simulink model "REAL_TIME_TRACKING"  (R2024b)
settings: Solver=ode4  StartTime=0.0  StopTime=T_SIM  FixedStep=T_s  RelTol=1e-3
undefined symbols (not defined in the file): control_par, controller_index, d, D, d_actual, H_enc, H_gyro, H_motion_cap, omega_M, omega_max, P_INIT_EKF, p_loss, PHI_INIT, Q_INIT, Q_INIT_LOC, r, R_3, r_actual, state_type, T_s, T_trj, trj_index, X, Y, Z_INIT_EKF
libraries: robotlib x6, sharedtransform x1
settings Model: Creator=llp  LastModifiedBy=tomailoren
settings OptimizationCC: DefaultParameterBehavior=Inlined  EnhancedBackFolding=on  PassReuseOutputArgsAs=Individual arguments  ZeroExternalMemoryAtStartup=off  ZeroInternalMemoryAtStartup=off  MaxStackSize=64  OptimizeBlockOrder=speed  DifferentSizesBufferReuse=on  OptimizationCustomize=off  EfficientTunableParamExpr=on
settings DebuggingCC: ParameterTunabilityLossMsg=error
settings SFSimCC: MATLABDynamicMemAlloc=off
settings RTWCC: Description=Embedded Coder  SystemTargetFile=ert.tlc  HardwareBoard=Robot Operating System 2 (ROS 2)  TLCOptions="-aInlineSetEventsForThisBaseRateFcn=TLC_FALSE -aSuppressMultiTaskScheduler=TLC_FALSE  -aRateBasedStepFcn=0"  TemplateMakefile=ert_default_tmf  Toolchain=Colcon Tools  TargetLang=C++
settings CodeAppCC: ForceParamTrailComments=on  IgnoreCustomStorageClasses=off  OperatorAnnotations=on  SimulinkDataObjDesc=on  SFDataObjDesc=on  InsertBlockDesc=on
settings ERTTargetCC: CodeInterfacePackaging=C++ class  RootIOFormat=Structure reference

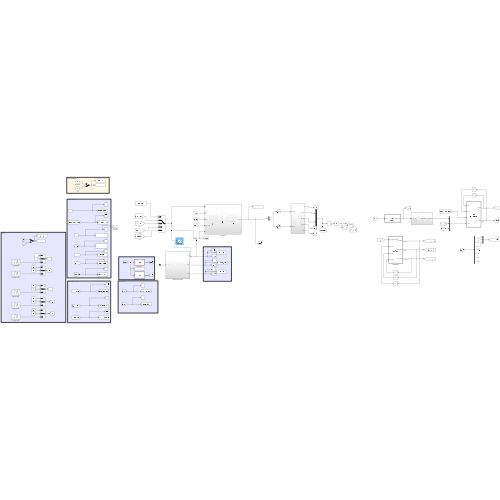
[thumbnail: Simulink's stored preview of the top-level diagram]
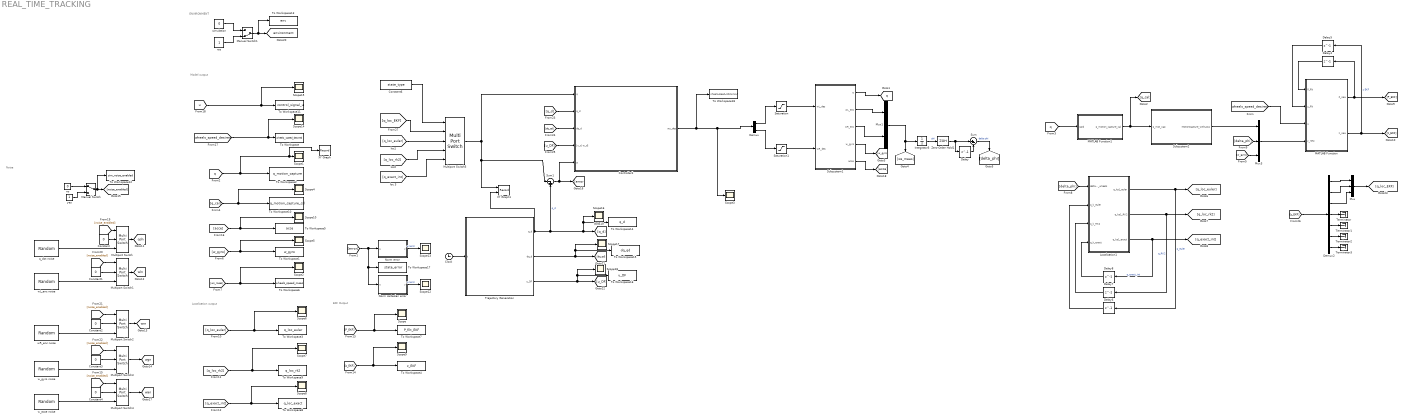
== system REAL_TIME_TRACKING ==
  note: Noise
  note: Localization output
  note: EKF Output
  note: Model output
  note: ENVIRONMENT
  Clock : Clock
  Constant{,1..4} (5 alike) : Constant  Value=0
  Constant6 : Constant  Value=state_type
  Controller1 : Subsystem
  Delay : Delay  DelayLength=1  InitialCondition=[0;0]  SampleTime=T_s
  Delay4 : Delay  DelayLength=1  InitialCondition=P_INIT_EKF  SampleTime=T_s
  Delay5 : Delay  DelayLength=1  InitialCondition=Z_INIT_EKF  SampleTime=T_s
  Delay6 : Delay  DelayLength=1  InitialCondition=Q_INIT_LOC
  Delay7 : Delay  DelayLength=1  InitialCondition=Q_INIT_LOC
  Delay8 : Delay  DelayLength=1  InitialCondition=Q_INIT_LOC
  Demux : Demux  Outputs=2
  Demux2 : Demux  Outputs=7
  Integrator5 : Integrator  InitialCondition=PHI_INIT
  Localization1 : MATLAB Function  TreatAsAtomicUnit=on
  MATLAB Function : MATLAB Function  TreatAsAtomicUnit=on
  MATLAB Function1 : MATLAB Function  TreatAsAtomicUnit=on
  Manual Switch : ManualSwitch
  Manual Switch1 : ManualSwitch  CurrentSetting=0
  Multiport Switch{,1..4} (5 alike) : MultiPortSwitch  DataPortOrder=Zero-based contiguous  Inputs=2  zeroidx=on  SaturateOnIntegerOverflow=off  InputSameDT=off
  Multiport Switch5 : MultiPortSwitch  Inputs=4  SaturateOnIntegerOverflow=off  InputSameDT=off
  Mux : Mux  Inputs=3
  Mux1 : Mux  Inputs=2
  Mux3 : Mux  Inputs=3
  Norm cartesian error : MATLAB Function  TreatAsAtomicUnit=on
  Norm error : MATLAB Function  TreatAsAtomicUnit=on
  Saturation : Saturate  UpperLimit=omega_max  LowerLimit=-omega_max
  Saturation1 : Saturate  UpperLimit=omega_max  LowerLimit=-omega_max
  Scope{,1..10,12..18} (18 alike) : Scope
  Subsystem1 : Subsystem
  Subsystem2 : Subsystem
  Sum : Sum  Inputs=|+-
  Sum1 : Sum  Inputs=|-+
  Terminator{,1..3} (4 alike) : Terminator
  To Workspace : ToWorkspace  VariableName=wheels_speed_desired  SaveFormat=Structure With Time  SampleTime=-1
  To Workspace1 : ToWorkspace  VariableName=w_gyro  SaveFormat=Structure With Time  SampleTime=-1
  To Workspace10 : ToWorkspace  VariableName=q_motion_capture_cal  SaveFormat=Structure With Time  SampleTime=-1
  To Workspace11 : ToWorkspace  VariableName=control_signal_u  SaveFormat=Timeseries  SampleTime=-1
  To Workspace12 : ToWorkspace  VariableName=sim_noise_enabled  SaveFormat=Structure  SampleTime=-1
      settings: Save2DSignal=2-D array (concatenate along first dimension)
  To Workspace13 : ToWorkspace  VariableName=env  SaveFormat=Structure  SampleTime=-1
      settings: Save2DSignal=2-D array (concatenate along first dimension)
  To Workspace14 : ToWorkspace  VariableName=q_d  SaveFormat=Structure With Time  SampleTime=-1
  To Workspace15 : ToWorkspace  VariableName=dq_qd  SaveFormat=Structure With Time  SampleTime=-1
  To Workspace16 : ToWorkspace  VariableName=u_DF  SaveFormat=Structure With Time  SampleTime=-1
  To Workspace17 : ToWorkspace  VariableName=state_error  SaveFormat=Structure With Time  SampleTime=-1
  To Workspace18 : ToWorkspace  VariableName=wheels_speed_robot_input  SaveFormat=Structure With Time  SampleTime=-1
  To Workspace2 : ToWorkspace  VariableName=q_motion_capture  SaveFormat=Structure With Time  SampleTime=-1
  To Workspace3 : ToWorkspace  VariableName=q_loc_euler  SaveFormat=Structure With Time  SampleTime=-1
  To Workspace4 : ToWorkspace  VariableName=z_EKF  SaveFormat=Structure With Time  SampleTime=-1
  To Workspace5 : ToWorkspace  VariableName=acce  SaveFormat=Structure With Time  SampleTime=-1
  To Workspace6 : ToWorkspace  VariableName=wheels_speed_meas  SaveFormat=Structure With Time  SampleTime=-1
  To Workspace7 : ToWorkspace  VariableName=P_filt_EKF  SaveFormat=Structure With Time  SampleTime=-1
  To Workspace8 : ToWorkspace  VariableName=q_loc_exact  SaveFormat=Structure With Time  SampleTime=-1
  To Workspace9 : ToWorkspace  VariableName=q_loc_rk2  SaveFormat=Structure With Time  SampleTime=-1
  Trajectory Generation : Subsystem
  XY Graph : Record  FileSettingsInternal="{\"entries\":[{\"content\":{\"excelSettings\":{\"content\":{},\"type\":\"Streamout.ExcelSettings\"}},\"type\":\"Streamout.FileSettingStorage\",\"uuid\":\"\"}],\"packageUris\":[\"http:\\/\\/schema.mathworks.com\\/mf0\\/streamout_blocks\\/R2020a\"],\"version\":\"1.0\"}"  Layout=[1 1]  SignalsInternal="{\"entries\":[{\"content\":{\"signals\":[{\"content\":{\"blockPath\":[],\"dimensions\":[3,1],\"domain\":\"\",\"hasChildren\":true,\"lineColor\":\"#4dbeee\",\"lineWidth\":2,\"port\":1,\"sid\":[\"\"],\"signalID\":1,\"signalName\":\"From2\"},\"type\":\"RecordBlkView.Signal\",\"uuid\":\"\"},{\"content\":{\"blockPath\":[],\"channel\":[1,1],\"dimensions\":[3,1],\"domain\":\"\",\"lineColor\":\"#77ac30\",\"lineWidth\":2,\"parentID\":1,\"port\":1,\"sid\":[\"\"],\"signalID\":2,\"signalName\":\"From2\"},\"type\":\"RecordBlkView.Signal\",\"uuid\":\"\"},{\"content\":{\"blockPath\":[],\"channel\":[2,1],\"dimensions\":[3,1],\"domain\":\"\",\"lineColor\":\"#fe330a\",\"lineWidth\":2,\"parentID\":1,\"port\":1,\"sid\":[\"\"],\"signalID\":3,\"signalName\":\"From2\"},\"type\":\"RecordBlkView.Signal\",\"uuid\":\"\"},{\"content\":{\"blockPath\":[],\"channel\":[3,1],\"dimensions\":[3,1],\"domain\":\"\",\"lineColor\":\"#22b573\",\"lineWidth\":2,\"parentID\":1,\"port\":1,\"sid\":[\"\"],\"signalID\":4,\"signalName\":\"From2\"},\"type\":\"RecordBlkView.Signal\",\"uuid\":\"\"}]},\"type\":\"RecordBlkView.InputSignals\",\"uuid\":\"\"}],\"packageUris\":[\"http:\\/\\/schema.mathworks.com\\/mf0\\/streamout_blocks\\/R2020a\"],\"version\":\"1.0\"}"  VisualizationBindings="{\"xyplotplugin\":{\"info\":[{\"series\":[],\"subplotID\":1}]}}"  CompatibilityTag=XY
  XY Graph1 : Record  FileSettingsInternal="{\"entries\":[{\"content\":{\"excelSettings\":{\"content\":{},\"type\":\"Streamout.ExcelSettings\"}},\"type\":\"Streamout.FileSettingStorage\",\"uuid\":\"\"}],\"packageUris\":[\"http:\\/\\/schema.mathworks.com\\/mf0\\/streamout_blocks\\/R2020a\"],\"version\":\"1.0\"}"  Layout=[1 1]  SignalsInternal="{\"entries\":[{\"content\":{\"signals\":[{\"content\":{\"blockPath\":[],\"dimensions\":[3,1],\"domain\":\"\",\"hasChildren\":true,\"lineColor\":\"#0072bd\",\"lineWidth\":2,\"port\":1,\"sid\":[\"\"],\"signalID\":1,\"signalName\":\"Multiport\\nSwitch5\"},\"type\":\"RecordBlkView.Signal\",\"uuid\":\"\"},{\"content\":{\"blockPath\":[],\"channel\":[1,1],\"dimensions\":[3,1],\"domain\":\"\",\"lineColor\":\"#0072bd\",\"lineWidth\":2,\"parentID\":1,\"plots\":[ 1 ],\"port\":1,\"sid\":[\"\"],\"signalID\":2,\"signalName\":\"Multiport\\nSwitch5\"},\"type\":\"RecordBlkView.Signal\",\"uuid\":\"\"},{\"content\":{\"blockPath\":[],\"dimensions\":[3,1],\"domain\":\"\",\"hasChildren\":true,\"lineColor\":\"#edb120\",\"lineWidth\":2,\"port\":2,\"sid\":[\"\"],\"signalID\":3,\"signalName\":\"q_d\"},\"type\":\"RecordBlkView.Signal\",\"uuid\":\"\"},{\"content\":{\"blockPath\":[],\"channel\":[1,1],\"dimensions\":[3,1],\"domain\":\"\",\"lineColor\":\"#d95319\",\"lineWidth\":2,\"parentID\":3,\"plots\":[ 1 ],\"port\":2,\"sid\":[\"\"],\"signalID\":4,\"signalName\":\"q_d\"},\"type\":\"RecordBlkView.Signal\",\"uuid\":\"\"},{\"content\":{\"blockPath\":[],\"channel\":[2,1],\"dimensions\":[3,1],\"domain\":\"\",\"lineColor\":\"#0072bd\",\"lineWidth\":2,\"parentID\":1,\"plots\":[ 1 ],\"port\":1,\"sid\":[\"\"],\"signalID\":5,\"signalName\":\"Multiport\\nSwitch5\"},\"type\":\"RecordBlkView.Signal\",\"uuid\":\"\"},{\"content\":{\"blockPath\":[],\"channel\":[3,1],\"dimensions\":[3,1],\"domain\":\"\",\"lineColor\":\"#ff13a6\",\"lineWidth\":2,\"parentID\":1,\"port\":1,\"sid\":[\"\"],\"signalID\":6,\"signalName\":\"Multiport\\nSwitch5\"},\"type\":\"RecordBlkView.Signal\",\"uuid\":\"\"},{\"content\":{\"blockPath\":[],\"channel\":[2,1],\"dimensions\":[3,1],\"domain\":\"\",\"lineColor\":\"#fe330a\",\"lineWidth\":2,\"parentID\":3,\"plots\":[ 1 ],\"port\":2,\"sid\":[\"\"],\"signalID\":7,\"signalName\":\"q_d\"},\"type\":\"RecordBlkView.Signal\",\"uuid\":\"\"},{\"content\":{\"blockPath\":[],\"channel\":[3,1],\"dimensions\":[3,1],\"domain\":\"\",\"lineColor\":\"#22b573\",\"lineWidth\":2,\"parentID\":3,\"port\":2,\"sid\":[\"\"],\"signalID\":8,\"signalName\":\"q_d\"},\"type\":\"RecordBlkView.Signal\",\"uuid\":\"\"}]},\"type\":\"RecordBlkView.InputSignals\",\"uuid\":\"\"}],\"packageUris\":[\"http:\\/\\/schema.mathworks.com\\/mf0\\/streamout_blocks\\/R2020a\"],\"version\":\"1.0\"}"  VisualizationBindings="{\"xyplotplugin\":{\"info\":[{\"series\":[{\"bindingParametersList\":[{\"parameter\":\"X-Axis\",\"signalID\":4,\"signalName\":\"q_d(1,1)\"},{\"parameter\":\"Y-Axis\",\"signalID\":7,\"signalName\":\"q_d(2,1)\"}],\"seriesID\":0},{\"bindingParametersList\":[{\"parameter\":\"X-Axis\",\"signalID\":2,\"signalName\":\"Multiport\\nSwitch5(1,1)\"},{\"parameter\":\"Y-Axis\",\"signalID\":5,\"signalName\":\"Multiport\\nSwitch5(2,1)\"}],\"seriesID\":1}],\"subplotID\":1}]}}"  CompatibilityTag=XY
  Zero-Order Hold1 : ZeroOrderHold  SampleTime=T_s
  no : Constant  Value=0
  q_dot noise : RandomNumber  Variance=0.01  SampleTime=T_s
  ros : Constant
  simulation : Constant  Value=0
  wL_enc noise : RandomNumber  Variance=0.01  Seed=1  SampleTime=T_s
  wR_enc noise : RandomNumber  Variance=0.01  Seed=2  SampleTime=T_s
  w_acce noise : RandomNumber  Variance=0.01  Seed=3  SampleTime=T_s
  w_gyro noise : RandomNumber  Variance=0.01  Seed=3  SampleTime=T_s
  yes : Constant
  tag scope: environment=global, q=global, qdn=global, wan=global, wgn=global, wln=global, wrn=global
  wires:
  [z_EKF] -> Scope9/1, To Workspace4/1
  [error] -> To Workspace17/1, Norm cartesian error/1(u), Norm error/1(u)
  simulation/1 -> Manual Switch1/1
  q_dot noise/1 -> Multiport Switch/3
  Integrator5/1 -> Zero-Order Hold1/1  "phi"
  [u] -> Scope15/1, To Workspace11/1
  [noise_enabled] -> Multiport Switch2/1
  Zero-Order Hold1/1 -> Delay/1, Sum/1
  [q_loc_rk2] -> Scope7/1, To Workspace9/1
  [wheels_speed_desired] -> Scope14/1, To Workspace/1
  Subsystem1/3(wR_enc) -> Mux1/2
  Norm cartesian error/1(y) -> Scope12/1  "p norm"
  [q] -> MATLAB Function1/1(q4id)
  Sum1/1 -> Controller1/5(e), [error]
  Norm error/1(y) -> Scope13/1  "e norm"
  Manual Switch/1 -> To Workspace12/1, [noise_enabled]
  Constant3/1 -> Multiport Switch3/2
  Saturation1/1 -> Subsystem1/2(wR_des)
  Delay/1 -> Sum/2
  [noise_enabled] -> Multiport Switch3/1
  wR_enc noise/1 -> Multiport Switch2/3
  ros/1 -> Manual Switch1/2
  Sum/1 -> [delta_phi]  "delta phi"
  Multiport Switch2/1 -> [wrn]
  Multiport Switch/1 -> [qdn]
  Demux/2 -> Saturation1/1
  Subsystem1/2(wL_enc) -> Mux1/1
  Mux1/1 -> Integrator5/1, [ws_meas]
  no/1 -> Manual Switch/1
  Subsystem1/5(acce) -> [acce]
  Subsystem1/4(w_gyro) -> [w_gyro]
  [P_EKF] -> Scope/1, To Workspace7/1
  [delta_phi] -> Localization1/1(delta_angles_wheels)
  Subsystem1/1(q) -> [q]
  w_gyro noise/1 -> Multiport Switch3/3
  Constant4/1 -> Multiport Switch4/2
  [q_exact_int] -> Scope8/1, To Workspace8/1
  [q_loc_euler] -> Scope6/1, To Workspace3/1
  [acce] -> Scope10/1, To Workspace5/1
  Multiport Switch1/1 -> [wln]
  w_acce noise/1 -> Multiport Switch4/3
  [noise_enabled] -> Multiport Switch4/1
  [noise_enabled] -> Multiport Switch/1
  [q_cal] -> To Workspace10/1, Scope4/1
  Constant/1 -> Multiport Switch/2
  yes/1 -> Manual Switch/2
  [q] -> XY Graph/1, Scope1/1, To Workspace2/1
  Constant2/1 -> Multiport Switch2/2
  wL_enc noise/1 -> Multiport Switch1/3
  Demux/1 -> Saturation/1
  Multiport Switch3/1 -> [wgn]
  [ws_meas] -> Scope2/1, To Workspace6/1
  [noise_enabled] -> Multiport Switch1/1
  Constant1/1 -> Multiport Switch1/2
  Multiport Switch4/1 -> [wan]
  MATLAB Function1/1(q_motion_capture_cal) -> [q_cal], Subsystem2/1(q_mot_cap)
  [w_gyro] -> Scope5/1, To Workspace1/1
  Saturation/1 -> Subsystem1/1(wL_des)
  Localization1/3(q_kp1_exact) -> [q_exact_int], Delay8/1  "q_exact_int"
  [w_gyro] -> Mux3/3
  [delta_phi] -> Mux3/2
  MATLAB Function/1(P_new) -> [P_EKF], Delay4/1
  Delay5/1 -> MATLAB Function/2(z_filt)
  Delay4/1 -> MATLAB Function/1(P_filt)
  Manual Switch1/1 -> [environment], To Workspace13/1
  MATLAB Function/2(z_new) -> [z_EKF], Delay5/1  "z EKF"
  Mux3/1 -> MATLAB Function/4(y_new)
  [wheels_speed_desired] -> MATLAB Function/3(u)
  Delay6/1 -> Localization1/2(q_k_euler)
  Delay8/1 -> Localization1/4(q_k_exact)
  Localization1/1(q_kp1_euler) -> [q_loc_euler], Delay6/1  "q_euler"
  Localization1/2(q_kp1_RK2) -> [q_loc_rk2], Delay7/1  "q_RK2"
  Constant6/1 -> Multiport Switch5/1
  Delay7/1 -> Localization1/3(q_k_RK2)
  Subsystem2/1(MotionCapture_withLoss) -> Mux3/1
  [q_loc_EKF] -> Multiport Switch5/2
  [q_loc_euler] -> Multiport Switch5/3
  Trajectory Generation/1(q_d) -> XY Graph1/2, Sum1/2, Scope16/1, To Workspace14/1, [q_d]  "q_d"
  [q_d] -> Controller1/2(q_d)
  [dq_qd] -> Controller1/3(dq_d)
  [u_DF] -> Controller1/4("[v_d, w_d]")
  Trajectory Generation/2(dq_d) -> To Workspace15/1, Scope17/1, [dq_qd]
  Trajectory Generation/3(u_DF) -> To Workspace16/1, Scope18/1, [u_DF]
  Clock/1 -> Trajectory Generation/1(t)
  Controller1/1(ws_des) -> To Workspace18/1, Demux/1, Scope3/1
  [z_EKF] -> Demux2/1
  Demux2/1 -> Mux/1
  Demux2/2 -> Mux/2
  Demux2/3 -> Mux/3
  Mux/1 -> [q_loc_EKF]
  Demux2/4 -> Terminator/1
  Demux2/5 -> Terminator1/1
  Demux2/6 -> Terminator2/1
  Demux2/7 -> Terminator3/1
  [q_loc_rk2] -> Multiport Switch5/4
  [q_exact_int] -> Multiport Switch5/5
  Multiport Switch5/1 -> Controller1/1(q), XY Graph1/1, Sum1/1

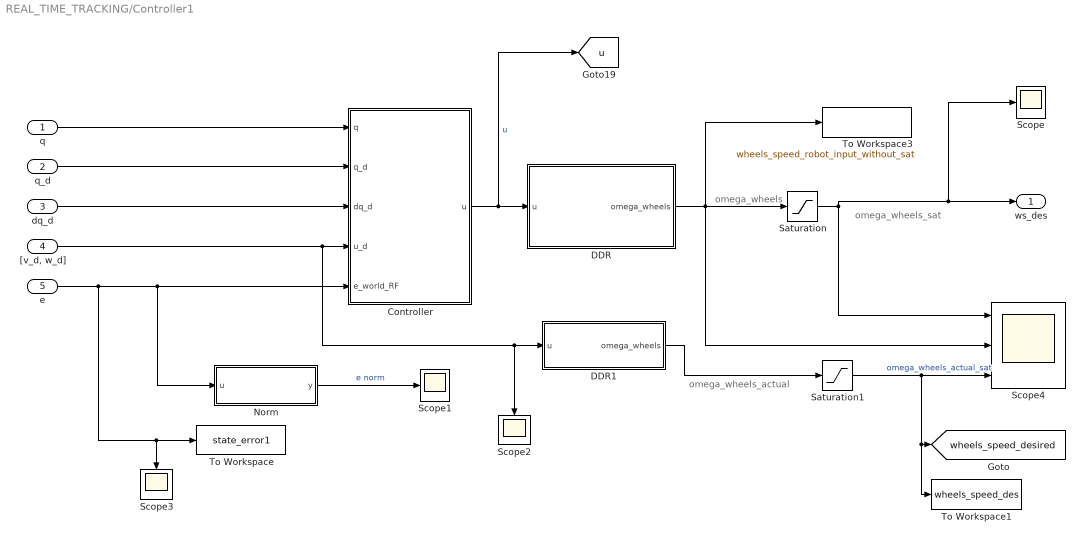
== system REAL_TIME_TRACKING/Controller1 ==
  note: omega_wheels_actual
  note: omega_wheels_sat
  note: omega_wheels
  q : Inport
  q_d : Inport  Port=2
  dq_d : Inport  Port=3
  "[v_d, w_d]" : Inport  Port=4
  e : Inport  Port=5
  Controller : MATLAB Function  TreatAsAtomicUnit=on
  DDR : MATLAB Function  TreatAsAtomicUnit=on
  DDR1 : MATLAB Function  TreatAsAtomicUnit=on
  Norm : MATLAB Function  TreatAsAtomicUnit=on
  Saturation : Saturate  UpperLimit=omega_M  LowerLimit=-omega_M
  Saturation1 : Saturate  UpperLimit=omega_M  LowerLimit=-omega_M
  Scope{,1..3} (4 alike) : Scope
  Scope4 : Scope  NumInputPorts=3
  To Workspace : ToWorkspace  VariableName=state_error1  SaveFormat=Structure With Time  SampleTime=-1
  To Workspace1 : ToWorkspace  VariableName=wheels_speed_des  SaveFormat=Structure With Time  SampleTime=-1
  To Workspace3 : ToWorkspace  VariableName=wheels_speed_robot_input_without_sat  SaveFormat=Structure With Time  SampleTime=-1
  ws_des : Outport
  tag scope: u=global, wheels_speed_desired=global
  wires:
  Saturation/1 -> Scope4/1, Scope/1, ws_des/1
  Saturation1/1 -> To Workspace1/1, [wheels_speed_desired], Scope4/3  "omega_wheels_actual_sat"
  DDR1/1(omega_wheels) -> Saturation1/1
  DDR/1(omega_wheels) -> To Workspace3/1, Scope4/2, Saturation/1
  q/1 -> Controller/1(q)
  dq_d/1 -> Controller/3(dq_d)
  Norm/1(y) -> Scope1/1  "e norm"
  q_d/1 -> Controller/2(q_d)
  e/1 -> Controller/5(e_world_RF), Norm/1(u), Scope3/1, To Workspace/1
  "[v_d, w_d]"/1 -> DDR1/1(u), Scope2/1, Controller/4(u_d)
  Controller/1(u) -> [u], DDR/1(u)  "u"

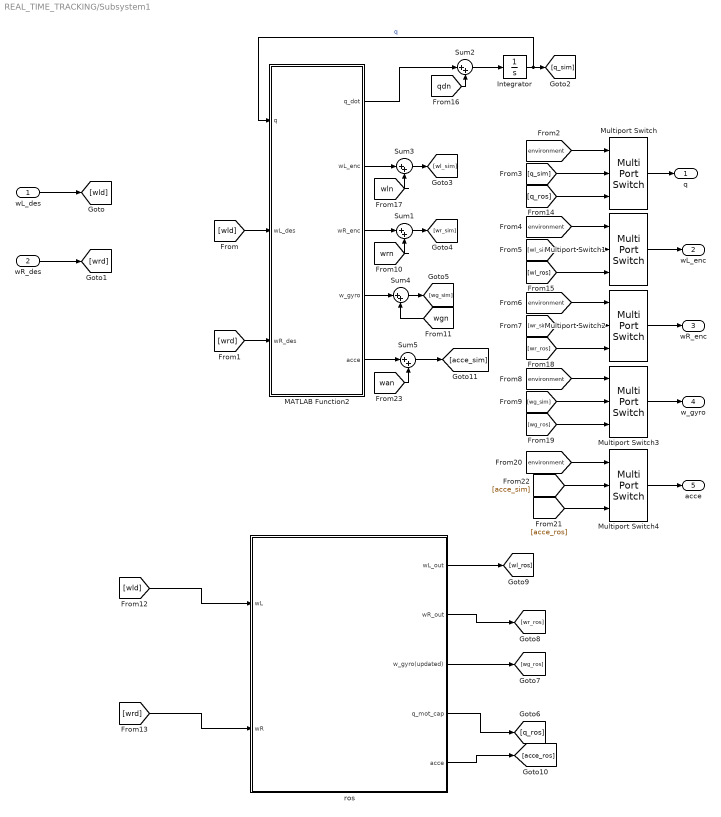
== system REAL_TIME_TRACKING/Subsystem1 ==
  wL_des : Inport
  wR_des : Inport  Port=2
  Integrator : Integrator  InitialCondition=Q_INIT
  MATLAB Function2 : MATLAB Function  TreatAsAtomicUnit=on
  Multiport Switch{,1..4} (5 alike) : MultiPortSwitch  DataPortOrder=Zero-based contiguous  Inputs=2  zeroidx=on  SaturateOnIntegerOverflow=off  InputSameDT=off
  Sum{1..5} (5 alike) : Sum  Inputs=|++
  ros : Subsystem
  q : Outport
  wL_enc : Outport  Port=2
  wR_enc : Outport  Port=3
  w_gyro : Outport  Port=4
  acce : Outport  Port=5
  wires:
  Sum2/1 -> Integrator/1
  Integrator/1 -> [q_sim], MATLAB Function2/1(q)  "q"
  [qdn] -> Sum2/2
  MATLAB Function2/1(q_dot) -> Sum2/1
  wL_des/1 -> [wld]
  wR_des/1 -> [wrd]
  [wld] -> MATLAB Function2/2(wL_des)
  [wrd] -> MATLAB Function2/3(wR_des)
  [environment] -> Multiport Switch/1
  [q_sim] -> Multiport Switch/2
  Multiport Switch/1 -> q/1
  [environment] -> Multiport Switch1/1
  [wl_sim] -> Multiport Switch1/2
  Multiport Switch1/1 -> wL_enc/1
  [environment] -> Multiport Switch2/1
  [wr_sim] -> Multiport Switch2/2
  Multiport Switch2/1 -> wR_enc/1
  [environment] -> Multiport Switch3/1
  [wg_sim] -> Multiport Switch3/2
  Multiport Switch3/1 -> w_gyro/1
  [wln] -> Sum3/2
  Sum3/1 -> [wl_sim]
  MATLAB Function2/2(wL_enc) -> Sum3/1
  [wrn] -> Sum1/2
  MATLAB Function2/3(wR_enc) -> Sum1/1
  Sum1/1 -> [wr_sim]
  [wgn] -> Sum4/2
  MATLAB Function2/4(w_gyro) -> Sum4/1
  Sum4/1 -> [wg_sim]
  [q_ros] -> Multiport Switch/3
  [wl_ros] -> Multiport Switch1/3
  [wr_ros] -> Multiport Switch2/3
  [wg_ros] -> Multiport Switch3/3
  Multiport Switch4/1 -> acce/1
  [environment] -> Multiport Switch4/1
  [acce_sim] -> Multiport Switch4/2
  [acce_ros] -> Multiport Switch4/3
  MATLAB Function2/5(acce) -> Sum5/1
  Sum5/1 -> [acce_sim]
  [wan] -> Sum5/2
  ros/1(wL_out) -> [wl_ros]
  ros/2(wR_out) -> [wr_ros]
  ros/5(acce) -> [acce_ros]
  ros/4(q_mot_cap) -> [q_ros]
  ros/3(w_gyro(updated)) -> [wg_ros]
  [wld] -> ros/1(wL)
  [wrd] -> ros/2(wR)

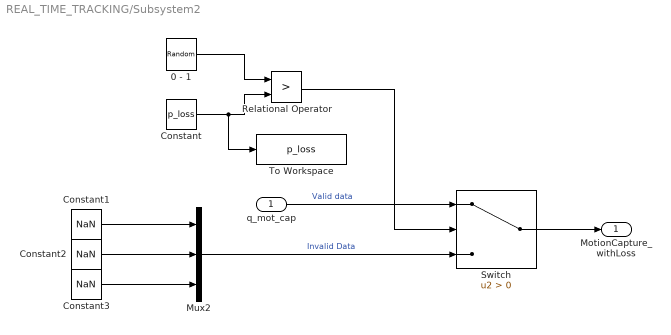
== system REAL_TIME_TRACKING/Subsystem2 ==
  q_mot_cap : Inport
  0 - 1 : UniformRandomNumber  Minimum=0  SampleTime=T_s
  Constant : Constant  Value=p_loss
  Constant1 : Constant  Value=NaN
  Constant2 : Constant  Value=NaN
  Constant3 : Constant  Value=NaN
  Mux2 : Mux  Inputs=3
  Relational Operator : RelationalOperator  Operator=>  OutDataTypeStr=boolean  RndMeth=Simplest  InputSameDT=off
  Switch : Switch  Criteria=u2 > Threshold  SaturateOnIntegerOverflow=off  InputSameDT=off
  To Workspace : ToWorkspace  VariableName=p_loss  SaveFormat=Structure  SampleTime=-1
      settings: Save2DSignal=2-D array (concatenate along first dimension)
  MotionCapture_withLoss : Outport
  wires:
  0 - 1/1 -> Relational Operator/1
  Constant/1 -> To Workspace/1, Relational Operator/2
  Switch/1 -> MotionCapture_withLoss/1
  Relational Operator/1 -> Switch/2
  Constant2/1 -> Mux2/2
  Mux2/1 -> Switch/3  "Invalid Data"
  Constant1/1 -> Mux2/1
  q_mot_cap/1 -> Switch/1  "Valid data"
  Constant3/1 -> Mux2/3

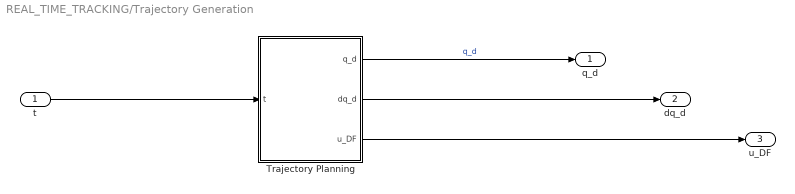
== system REAL_TIME_TRACKING/Trajectory Generation ==
  t : Inport
  Trajectory Planning : MATLAB Function  TreatAsAtomicUnit=on
  q_d : Outport
  dq_d : Outport  Port=2
  u_DF : Outport  Port=3
  wires:
  Trajectory Planning/1(q_d) -> q_d/1  "q_d"
  Trajectory Planning/2(dq_d) -> dq_d/1
  Trajectory Planning/3(u_DF) -> u_DF/1
  t/1 -> Trajectory Planning/1(t)

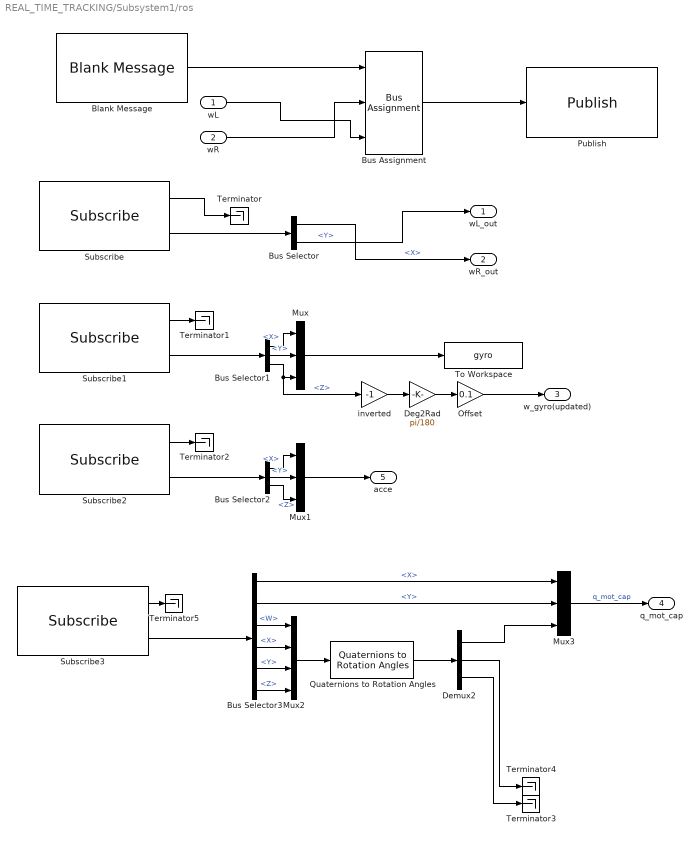
== system REAL_TIME_TRACKING/Subsystem1/ros ==
  wL : Inport
  wR : Inport  Port=2
  Blank Message : robotlib/Blank Message  messageClass=Message  entityType=geometry_msgs/Vector3  messageType=geometry_msgs/Vector3  SampleTime=T_s  legacyBusStruct=off
  Bus Assignment : BusAssignment  AssignedSignals=X,Y
  Bus Selector : BusSelector  OutputSignals=X,Y
  Bus Selector1 : BusSelector  OutputSignals=X,Y,Z
  Bus Selector2 : BusSelector  OutputSignals=X,Y,Z
  Bus Selector3 : BusSelector  OutputSignals=Pose.Pose.Position.X,Pose.Pose.Position.Y,Pose.Pose.Orientation.W,Pose.Pose.Orientation.X,Pose.Pose.Orientation.Y,Pose.Pose.Orientation.Z
  Deg2Rad : Gain  Gain=pi/180
  Demux2 : Demux  Outputs=3
  Mux : Mux  Inputs=3
  Mux1 : Mux  Inputs=3
  Mux2 : Mux
  Mux3 : Mux  Inputs=3
  Offset : Gain  Gain=0.1
  Publish : robotlib/Publish  topicSource=Select from ROS network  topic=/turtlebot_01/cmd_wheels  messageType=geometry_msgs/Vector3  legacyBusStruct=off  messageQueueLength=1
  Quaternions to Rotation Angles : sharedtransform/Quaternions to Rotation Angles  rotationOrder=ZYX  aMode=aMode
  Subscribe : robotlib/Subscribe  topicSource=Select from ROS network  topic=/turtlebot_01/wheelSpeeds  messageType=geometry_msgs/Vector3  SampleTime=T_s  legacyBusStruct=off  messageQueueLength=1
  Subscribe1 : robotlib/Subscribe  topicSource=Select from ROS network  topic=/turtlebot_01/gyroscope  messageType=geometry_msgs/Vector3  SampleTime=T_s  legacyBusStruct=off  messageQueueLength=1
  Subscribe2 : robotlib/Subscribe  topicSource=Select from ROS network  topic=/turtlebot_01/accelerometer  messageType=geometry_msgs/Vector3  SampleTime=T_s  legacyBusStruct=off  messageQueueLength=1
  Subscribe3 : robotlib/Subscribe  topicSource=Select from ROS network  topic=/turtlebot_01/odom  messageType=nav_msgs/Odometry  SampleTime=T_s  legacyBusStruct=off  messageQueueLength=1
  Terminator{,1..5} (6 alike) : Terminator
  To Workspace : ToWorkspace  VariableName=gyro  SaveFormat=Structure With Time  SampleTime=-1
  inverted : Gain  Gain=-1
  wL_out : Outport
  wR_out : Outport  Port=2
  w_gyro(updated) : Outport  Port=3
  q_mot_cap : Outport  Port=4
  acce : Outport  Port=5
  wires:
  Subscribe2/2 -> Bus Selector2/1
  Bus Selector3/6 -> Mux2/4  "<Z>"
  Mux3/1 -> q_mot_cap/1  "q_mot_cap"
  wR/1 -> Bus Assignment/2
  Bus Selector/1 -> wR_out/1  "<X>"
  Bus Selector1/2 -> Mux/2  "<Y>"
  Bus Selector2/2 -> Mux1/2  "<Y>"
  Bus Selector2/1 -> Mux1/1  "<X>"
  Bus Assignment/1 -> Publish/1
  Subscribe2/1 -> Terminator2/1
  Demux2/2 -> Terminator4/1
  Mux2/1 -> Quaternions to Rotation Angles/1
  inverted/1 -> Deg2Rad/1
  Bus Selector3/4 -> Mux2/2  "<X>"
  Bus Selector3/1 -> Mux3/1  "<X>"
  Subscribe3/1 -> Terminator5/1
  Subscribe/2 -> Bus Selector/1
  Mux1/1 -> acce/1
  Deg2Rad/1 -> Offset/1
  Bus Selector3/5 -> Mux2/3  "<Y>"
  Quaternions to Rotation Angles/1 -> Demux2/1
  Bus Selector1/3 -> inverted/1, Mux/3  "<Z>"
  Demux2/3 -> Terminator3/1
  Demux2/1 -> Mux3/3
  Offset/1 -> w_gyro(updated)/1
  wL/1 -> Bus Assignment/3
  Bus Selector3/3 -> Mux2/1  "<W>"
  Bus Selector1/1 -> Mux/1  "<X>"
  Subscribe3/2 -> Bus Selector3/1
  Bus Selector2/3 -> Mux1/3  "<Z>"
  Mux/1 -> To Workspace/1
  Subscribe/1 -> Terminator/1
  Bus Selector/2 -> wL_out/1  "<Y>"
  Subscribe1/2 -> Bus Selector1/1
  Subscribe1/1 -> Terminator1/1
  Blank Message/1 -> Bus Assignment/1
  Bus Selector3/2 -> Mux3/2  "<Y>"

== matlab function REAL_TIME_TRACKING/Norm cartesian error ==
  data: u input; y output
function y = fcn(u)

y = sqrt(sum(u(1:2).^2));

== matlab function REAL_TIME_TRACKING/Norm error ==
  data: u input; y output
function y = fcn(u)
y = [u(1);u(2); wrapToPi(u(3))];

== matlab function REAL_TIME_TRACKING/Controller1/Norm ==
  data: u input; y output
function y = fcn(u)

y = sqrt(sum(u(1:2).^2));

== matlab function REAL_TIME_TRACKING/Controller1/DDR ==
  data: u input; omega_wheels output; r parameter; d parameter
function omega_wheels = kin2omegawheels(u, r, d)
omega_l = u(1)/r-d/(2*r)*u(2);
omega_r = u(1)/r+d/(2*r)*u(2);
omega_wheels = [omega_l;omega_r];

== matlab function REAL_TIME_TRACKING/Controller1/DDR1 ==
  data: u input; omega_wheels output; r_actual parameter; d_actual parameter
function omega_wheels = kin2omegawheels(u, r_actual, d_actual)
omega_l = u(1)/r_actual-d_actual/(2*r_actual)*u(2);
omega_r = u(1)/r_actual+d_actual/(2*r_actual)*u(2);
omega_wheels = [omega_l;omega_r];

== matlab function REAL_TIME_TRACKING/Localization1 ==
  data: delta_angles_wheels input; q_k_euler input; q_k_RK2 input; q_k_exact input; r_actual parameter; d_actual parameter; q_kp1_euler output; T_s parameter; q_kp1_RK2 output; q_kp1_exact output
function [q_kp1_euler, q_kp1_RK2, q_kp1_exact] = localization(delta_angles_wheels, q_k_euler, q_k_RK2, q_k_exact, r_actual, d_actual, T_s)

    r = r_actual;
    d = d_actual;

    % extraction data
    delta_phi_L = delta_angles_wheels(1);
    delta_phi_R = delta_angles_wheels(2);

    x_k_euler = q_k_euler(1); 
    y_k_euler = q_k_euler(2); 
    theta_k_euler = q_k_euler(3);
    
    x_k_RK2 = q_k_RK2(1); 
    y_k_RK2 = q_k_RK2(2); 
    theta_k_RK2 = q_k_RK2(3);

    x_k_exact = q_k_exact(1);
    y_k_exact = q_k_exact(2); 
    theta_k_exact = q_k_exact(3);


    % velocities estimate
    v_k = r / (2*T_s) * (delta_phi_R + delta_phi_L);
    w_k = r / (d*T_s) * (delta_phi_R - delta_phi_L);
    
    % Euler integration
    x_kp1_euler = x_k_euler + v_k * T_s * cos(theta_k_euler);
    y_kp1_euler = y_k_euler + v_k * T_s * sin(theta_k_euler);
    theta_kp1_euler = theta_k_euler + w_k * T_s;
    
    q_kp1_euler = [x_kp1_euler; y_kp1_euler; theta_kp1_euler];
    
    % RK2 Integration
    x_kp1_RK2 = x_k_RK2 + v_k * T_s * cos(theta_k_RK2 + (w_k * T_s)/2);
    y_kp1_RK2 = y_k_RK2 + v_k * T_s * sin(theta_k_RK2 + (w_k * T_s)/2);
    theta_kp1_RK2 = theta_k_RK2 + w_k * T_s;
    
    q_kp1_RK2 = [x_kp1_RK2; y_kp1_RK2; theta_kp1_RK2];
    
    % Exact Integration
    if abs(w_k) < 1e-4
        % use RK2 approximation to avoid division by zero when w_k is near 0
        x_kp1_exact = x_k_exact + v_k * T_s * cos(theta_k_exact + (w_k * T_s)/2);
        y_kp1_exact = y_k_exact + v_k * T_s * sin(theta_k_exact + (w_k * T_s)/2);
    else
        % Exact formulas
        x_kp1_exact = x_k_exact + (v_k / w_k) * (sin(theta_k_exact + w_k * T_s) - sin(theta_k_exact));
        y_kp1_exact = y_k_exact - (v_k / w_k) * (cos(theta_k_exact + w_k * T_s) - cos(theta_k_exact));
    end
    theta_kp1_exact = theta_k_exact + w_k * T_s;
    
    q_kp1_exact = [x_kp1_exact; y_kp1_exact; theta_kp1_exact];
    
end

== matlab function REAL_TIME_TRACKING/MATLAB Function1 ==
  data: q4id input; q_motion_capture_cal output
function q_motion_capture_cal = calibration(q4id)

x_off_cal = -0.00434;
y_off_cal = -0.00361;
theta_off = 0.02331;


theta_cal = q4id(3) - theta_off;
x_cal = q4id(1) - (x_off_cal * cos(theta_cal) - y_off_cal * sin(theta_cal));
y_cal = q4id(2) - (x_off_cal * sin(theta_cal) + y_off_cal * cos(theta_cal));


q_motion_capture_cal = [x_cal; y_cal; theta_cal];

== matlab function REAL_TIME_TRACKING/Subsystem1/MATLAB Function2 ==
  data: q input; q_dot output; wL_des input; wR_des input; wL_enc output; wR_enc output; w_gyro output; r parameter; d parameter; T_s parameter; acce output
function [q_dot, wL_enc, wR_enc, w_gyro, acce] = robot_simulator(q, wL_des, wR_des, r, d, T_s)
    
    wL_enc = wL_des;
    wR_enc = wR_des;
      
    v = (r/2) * (wR_des + wL_des);
    omega = (r/d) * (wR_des - wL_des);
    
    w_gyro = -omega;
    
    q_dot= zeros(3,1);
    
    q_dot(1) = v*cos(q(3));
    q_dot(2) = v*sin(q(3));
    q_dot(3) = omega;

    acce = [0;0;0];
    
end

== matlab function REAL_TIME_TRACKING/Trajectory Generation/Trajectory Planning ==
  data: t input; q_d output; dq_d output; u_DF output; trj_index parameter; T_trj parameter
function [q_d, dq_d, u_DF] = get_trj(t, trj_index, T_trj)
if trj_index == 1
    % line
    vel = 1/T_trj;
    q_d = [0; vel*t; pi/2];
    dq_d = [0; vel; 0];
    u_DF = [vel; 0];
elseif trj_index == 2
    % circle
    r = 0.5;
    omega = 2*pi/T_trj;
    theta_prime = omega*t;
    q_d = [r*cos(theta_prime); r*sin(theta_prime); theta_prime + pi/2];
    dq_d = [-omega*r*sin(theta_prime); omega*r*cos(theta_prime); omega];
    u_DF = [omega*r; omega];
elseif trj_index == 3
    %  square
    T_cycle = mod(t, T_trj);
    side_length = 1;
    vel = side_length/(T_trj/4);
    if T_cycle<=T_trj/4
        t_side = T_cycle;
        q_d = [0;  t_side*vel; pi/2];
        dq_d = [0;vel;0];
        u_DF = [vel; 0];
    elseif T_cycle <=T_trj/2
        t_side = T_cycle - T_trj/4;
        q_d = [-vel*t_side; side_length ;pi];
        dq_d = [-vel;0;0];
        u_DF = [vel;0];
    elseif T_cycle <= 3*T_trj/4
        t_side = T_cycle - T_trj/2;
        q_d = [-side_length; side_length-vel*t_side; -pi/2];
        dq_d = [0;-vel;0];
        u_DF = [vel;0];
    else
        t_side = T_cycle - 3*T_trj/4;
        q_d = [-side_length + vel*t_side; 0; 0];
        dq_d = [vel;0;0];
        u_DF = [vel;0];
    end
elseif trj_index == 4
    % 8-shape
    R = 0.4;
    omega = 2*pi/T_trj;
    x_d = R*sin(2*omega*t);
    dx_d = R*2*omega*cos(2*omega*t);
    ddx_d = -R*4*omega.^2*sin(2*omega*t);
    y_d = R*sin(omega*t);
    dy_d = R*omega*cos(omega*t);
    ddy_d = -R*omega.^2*sin(omega*t);
    theta_d = atan2(dy_d, dx_d);
    dtheta_d = (dx_d*ddy_d -  dy_d*ddx_d)/(dx_d.^2+dy_d.^2);
    q_d = [x_d;y_d;theta_d];
    dq_d = [dx_d;dy_d;dtheta_d];
    u_DF = [sqrt(dx_d.^2 + dy_d.^2);dtheta_d];


elseif trj_index == 5
    % S cartesian traj
    
    %% --- Parametri traiettoria
    Ta = 1;
    Tc = 10;
    qi = [-0.5; -0.5; pi/2];
    qf = [ 0.5;  0.5; pi/2];
    ki = 4;
    kf = 4;
    
    %% --- Time Law Trapezoidale (scalare in t) ---
    vc = 1 / (Ta + Tc);
    a  = vc / Ta;
    T_end = 2*Ta + Tc;
    
    if t < Ta
        % Fase 1: accelerazione
        s_dot = a * t;
        s     = 0.5 * a * t^2;
    elseif t < (Ta + Tc)
        % Fase 2: velocità costante
        s_dot = vc;
        s     = 0.5 * a * Ta^2 + vc * (t - Ta);
    elseif t < T_end
        % Fase 3: decelerazione
        dt3   = t - Ta - Tc;
        s_dot = vc - a * dt3;
        s     = 0.5*a*Ta^2 + vc*Tc + vc*dt3 - 0.5*a*dt3^2;
    else
        % Fase 4: fine traiettoria
        s_dot = 0;
        s     = 1;
    end
    
    %% --- Polinomi Cubici ---
    xi = qi(1); yi = qi(2); thetai = qi(3);
    xf = qf(1); yf = qf(2); thetaf = qf(3);
    
    coeff_a = [xf,  xi,  kf*cos(thetaf) - 3*xf,  ki*cos(thetai) + 3*xi];
    coeff_b = [yf,  yi,  kf*sin(thetaf) - 3*yf,  ki*sin(thetai) + 3*yi];
    
    % Posizione geometrica
    x_s = coeff_a(1)*s^3 - coeff_a(2)*(s^3-3*s^2+3*s-1) ...
        + coeff_a(3)*(s^3-s^2) + coeff_a(4)*(s^3-2*s^2+s);
    y_s = coeff_b(1)*s^3 - coeff_b(2)*(s^3-3*s^2+3*s-1) ...
        + coeff_b(3)*(s^3-s^2) + coeff_b(4)*(s^3-2*s^2+s);
    
    % Prima derivata rispetto a s
    x_ds = 3*coeff_a(1)*s^2 - coeff_a(2)*(3*s^2-6*s+3) ...
         + coeff_a(3)*(3*s^2-2*s) + coeff_a(4)*(3*s^2-4*s+1);
    y_ds = 3*coeff_b(1)*s^2 - coeff_b(2)*(3*s^2-6*s+3) ...
         + coeff_b(3)*(3*s^2-2*s) + coeff_b(4)*(3*s^2-4*s+1);
    
    % Seconda derivata rispetto a s
    x_dds = 6*coeff_a(1)*s - coeff_a(2)*(6*s-6) + coeff_a(3)*(6*s-2) + coeff_a(4)*(6*s-4);
    y_dds = 6*coeff_b(1)*s - coeff_b(2)*(6*s-6) + coeff_b(3)*(6*s-2) + coeff_b(4)*(6*s-4);
    
    %% --- Input geometrici ---
    v_tilde     = sqrt(x_ds^2 + y_ds^2);
    omega_tilde = (x_ds * y_dds - y_ds * x_dds) / (x_ds^2 + y_ds^2);
    
    %% --- Input reali (feedforward) ---
    v = v_tilde * s_dot;
    w = omega_tilde * s_dot;

    u_DF = [v;w];
    
    %% --- Stato desiderato q_d = [x; y; theta] ---
    theta_d = atan2(y_ds, x_ds);   % orientamento tangente alla curva
    q_d  = [x_s; y_s; theta_d];
    
    %% --- Velocità desiderata dq_d = [dx; dy; dtheta] ---
    % Per un unicycle: dx = v*cos(theta), dy = v*sin(theta), dtheta = w
    dq_d = [v * cos(theta_d);
            v * sin(theta_d);
            w];
else
    q_d = [0;0;0];
    dq_d = [0;0;0];
    u_DF = [0;0];
end

== matlab function REAL_TIME_TRACKING/MATLAB Function ==
  data: P_filt input; P_new output; z_filt input; z_new output; u input; y_new input; D parameter; T_s parameter; r_actual parameter; d_actual parameter; H_enc parameter; H_gyro parameter; H_motion_cap parameter; R_3 parameter
function [P_new, z_new] = EKF_filtering(P_filt, z_filt, u, y_new, D, T_s, r_actual, d_actual, H_enc, H_gyro, H_motion_cap, R_3)

    % Def state z_filt: [xk , yk , thetak , delta_phi_L_km1 , delta_phi_R_km1 , wLk , wRk ]

    r = r_actual;
    d = d_actual;
        
    % Extraction variables
    x_k = z_filt(1);
    y_k = z_filt(2);
    theta_k = z_filt(3);
    delta_phi_L_km1 = z_filt(4);
    delta_phi_R_km1 = z_filt(5); 
    wL_k = z_filt(6);               % estimate wheels velocities
    wR_k = z_filt(7);
    
    uL_k = u(1);                    % actual wheels velocities (from command input v,w)
    uR_k = u(2);

    % ----------------------

    % PREDICT STEP
    v_k = (r/2) * (wL_k + wR_k);
    omega_k = (r/d) * (wR_k - wL_k);
    theta_mean = theta_k + (omega_k * T_s) / 2;
        
    % State Prediction (approximation with RK2)
    x_kp1 = x_k + v_k * T_s * cos(theta_mean);
    y_kp1 = y_k + v_k * T_s * sin(theta_mean);
    theta_kp1 = theta_k + omega_k * T_s;
    
    delta_phi_L_k = wL_k * T_s;
    delta_phi_R_k = wR_k * T_s;
    
    wL_kp1 = uL_k; 
    wR_kp1 = uR_k;
    
    z_hat = [x_kp1; y_kp1; theta_kp1; delta_phi_L_k; delta_phi_R_k; wL_kp1; wR_kp1];
    
    % F derivation
    F = zeros(7,7);
    
    F(1,1) = 1;
    F(1, 3) = -T_s * v_k * sin(theta_mean);
    F(1, 6) = (T_s * r / 2) * cos(theta_mean) - v_k * T_s * sin(theta_mean) * (-T_s * r / (2 * d));
    F(1, 7) = (T_s * r / 2) * cos(theta_mean) - v_k * T_s * sin(theta_mean) * (T_s * r / (2 * d));
    
    F(2,2) = 1;
    F(2, 3) = v_k * T_s * cos(theta_mean);
    F(2, 6) = (T_s * r / 2) * sin(theta_mean) + v_k * T_s * cos(theta_mean) * (-T_s * r / (2 * d));
    F(2, 7) = (T_s * r / 2) * sin(theta_mean) + v_k * T_s * cos(theta_mean) * (T_s * r / (2 * d));

    F(3,3) = 1;
    F(3, 6) = -T_s * r / d;
    F(3, 7) = T_s * r / d;

    F(4, 6) = T_s;
    F(5, 7) = T_s;
    
    % Covariance Prediction
    P_hat = F * P_filt * F' + D;
    
    % ----------------------

    % UPDATE STEP
    % H and R will depend on the measurement data y_new and Test_case

    % enc_values (delta_phi)
    % IMU_values (w_gyro)
    % Motion_capture (state q)

    % y_new = [x; y; theta; delta_phi_L; delta_phi_R; omega_gyro]

    %% OBSERVATION MATRIX H ALWAYS FULL (6X7) AND ALSO Y_NEW (6X1) 
    H_full = [H_motion_cap; H_enc; H_gyro];
    y_meas = y_new; 
    
    % Start with full matrix R_3 
    R_current = R_3;
    INFINITY_VAR = 1e9; % Infinite var to put down the Kalman gain

    % IMU not available
    R_current(6,6) = INFINITY_VAR;
    
    % TEST 3: all active, possibile data loss
    if any(isnan(y_new(1:3)))   
        y_meas(1:3) = 0;    % force to zero just for completness
        R_current(1,1) = INFINITY_VAR; 
        R_current(2,2) = INFINITY_VAR; 
        R_current(3,3) = INFINITY_VAR;
    end

    
    % Innovation e_pred
    y_hat = H_full * z_hat;
    e_kp1 = y_meas - y_hat;
    
    % Kalman Gain K_pred
    K = P_hat * H_full' / (H_full * P_hat * H_full' + R_current);   
    
    % State and Covariance Update
    z_new = z_hat + K * e_kp1;
    P_new = P_hat - K * H_full * P_hat;


end

== matlab function REAL_TIME_TRACKING/Controller1/Controller ==
  data: q input; q_d input; dq_d input; u_d input; u output; e_world_RF input; controller_index parameter; control_par parameter
function u = fcn(q, q_d, dq_d, u_d, e_world_RF, controller_index, control_par)

    % LINREAR controller
    if controller_index == 1
                
        vd = u_d(1); wd = u_d(2);

        % derive control matrix K
        K = linear_gains(control_par, vd, wd);
        k1 = K(1); k2 = K(2); k3 = K(3);

        % rotation of the error
        e_body = error_rotation(e_world_RF, q);
        e1 = e_body(1); e2 = e_body(2); e3 = e_body(3); 
    
        % Linear Contrl Law
        % Define u_aux_1, u_aux_2 auxiliar inputs
        u1_aux = -k1 * e1;
        u2_aux = -k2 * e2 - k3 * e3;
        
        % 3. Real model inputs    
        v = vd * cos(e3) - u1_aux;
        w = wd - u2_aux;
        
        % Saturation (if i want a saturation directly on v and w
        % v = max(min(v, 1.5), -1.5); 
        % w = max(min(w, 3.0), -3.0);
        
        u = [v; w];


    % --------------------------------------
    % NON LINEAR controller
    elseif controller_index == 2
        
        vd = u_d(1); wd = u_d(2);

        % derive control matrix K
        K = NL_gains(control_par, vd, wd);
        k1 = K(1); k2 = K(2); k3 = K(3); 

        % rotation of the error
        e_body = error_rotation(e_world_RF, q);
        e1 = e_body(1); e2 = e_body(2); e3 = e_body(3); 
    
        % NON-Linear Contrl Law
        
        % Singularity: sinc(e3) = sin(e3)/e3
        if abs(e3) < 1e-4
            sinc_e3 = 1;
        else
            sinc_e3 = sin(e3)/e3;
        end
        
        % Define u_aux_1, u_aux_2 auxiliar inputs
        u1_aux = -k1 * e1;
        u2_aux = -k2 * vd * sinc_e3 * e2 - k3 * e3;
       
        % Real model inputs
        v = vd * cos(e3) - u1_aux;
        w = wd - u2_aux;
        
        % Saturation  
        % v = max(min(v, 1.5), -1.5); 
        % w = max(min(w, 3.0), -3.0);
        
        u = [v; w];


    % --------------------------------------
    % FEEDBACK LINEARIZATION (OUTPUT ERROR FB)
    elseif controller_index == 3
    % here it is considered q the B_point_q, the same for q_d and the error

        theta = q(3);
        k1 = control_par(1); k2 = control_par(2); b = control_par(3);

        % build K matrix
        K = [k1 , 0 ; 0 , k2];

        % I just need the the first 2 components of the error (ep_x, ep_y)
        % in the world frame
        ep = [ e_world_RF(1) ; e_world_RF(2) ];
  
        % same for the pose
        pBd_dot = [ dq_d(1) ; dq_d(2) ];
        
        T_inv = [cos(theta),       sin(theta);
                 -(1/b) * sin(theta), (1/b) * cos(theta)];
    
        u = T_inv * (pBd_dot + K * ep);     % u = [v; w]

    else
        u = u_d;
    end
end

% ------------------------------------------------------------------

% LOCAL FUNCTIONS


function e_body = error_rotation(e_w, q)

    % Extracts the current robot orientation
    theta = q(3);
    
    % Normalize the orientation error (3rd component) to be within [-pi, pi]
    % This prevents the robot from making unnecessary 360-degree turns.
    e_theta = e_w(3);
    e_w(3) = atan2(sin(e_theta), cos(e_theta));
    
    % Rotation matrix transpose
    R_T = [ cos(theta), sin(theta), 0;
           -sin(theta), cos(theta), 0;
                0,          0,      1];
            
    % Compute error in Body Frame
    e_body = R_T * e_w;

end
    
function K = linear_gains(control_par, vd, wd)
    xi = control_par(1);
    a = control_par(2);

    k1 = 2 * xi * a; 
    k3 = k1;
    
    % if vd is zero the gain will be huge (controlled then by saturation)
    if abs(vd) < 1e-4
        if vd >= 0
            vd = 1e-4;
        else
            vd = -1e-4;
        end
    end
        
    k2 = (a^2 - wd^2)/vd;

    K = [k1; k2; k3];
end


function K = NL_gains(control_par, vd, wd)
    xi = control_par(1);
    b = control_par(2);

    k1 = 2 * xi * sqrt(b*vd + wd^2); 
    k3 = k1;
    k2 = b;

    K = [k1; k2; k3];
end
